simulink model "Grp43_Model"  (R2023a)
settings: Solver=FixedStepAuto  StartTime=0.0  StopTime=10.0  FixedStep=1e-5  RelTol=1e-3
values from neighbouring files (symbols this model uses):
  g = 9.8    [Grp43_Code.m]    (also in Grp43_part2_code.m = 9.81; e01 2.m; grp43_asgn2_2.m)
  l = 0.36    [Grp43_Code.m]    (also in Grp43_part2_code.m; e01 2.m; grp43_asgn2_2.m)
  m = 0.26    [Grp43_Code.m]    (also in Grp43_part2_code.m; e01 2.m; grp43_asgn2_2.m)
  M = 2.4    [Grp43_Code.m]    (also in Grp43_part2_code.m; e01 2.m; grp43_asgn2_2.m)
settings Model: Creator=jitbi  LastModifiedBy=Anirvan Krishna

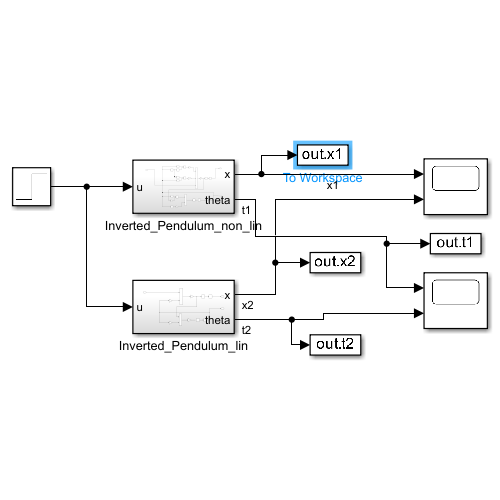
[thumbnail: Simulink's stored preview of the top-level diagram]
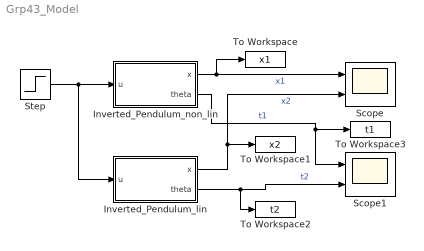
== system Grp43_Model ==
  Inverted_Pendulum_lin : Subsystem
  Inverted_Pendulum_non_lin : Subsystem
  Scope : Scope  NumInputPorts=2
  Scope1 : Scope  NumInputPorts=2
  Step : Step  Time=0
  To Workspace : ToWorkspace  VariableName=x1  SampleTime=-1
  To Workspace1 : ToWorkspace  VariableName=x2  SampleTime=-1
  To Workspace2 : ToWorkspace  VariableName=t2  SampleTime=-1
  To Workspace3 : ToWorkspace  VariableName=t1  SampleTime=-1
  wires:
  Step/1 -> Inverted_Pendulum_lin/1(u), Inverted_Pendulum_non_lin/1(u)
  Inverted_Pendulum_non_lin/1(x) -> Scope/1, To Workspace/1  "x1"
  Inverted_Pendulum_lin/1(x) -> To Workspace1/1, Scope/2  "x2"
  Inverted_Pendulum_non_lin/2(theta) -> To Workspace3/1, Scope1/1  "t1"
  Inverted_Pendulum_lin/2(theta) -> To Workspace2/1, Scope1/2  "t2"

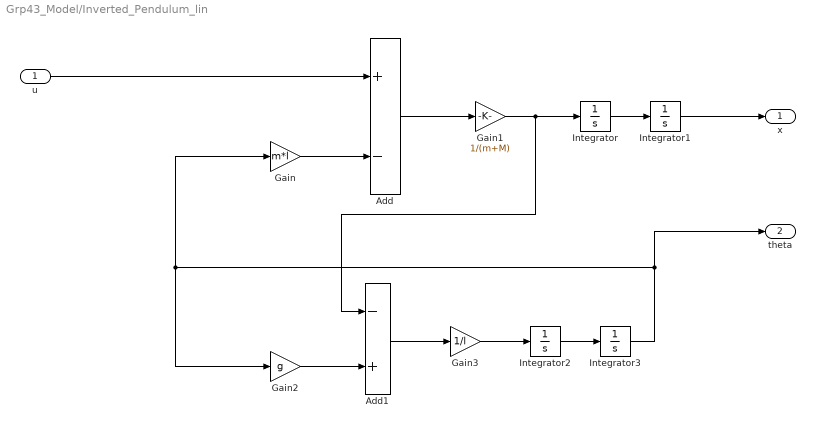
== system Grp43_Model/Inverted_Pendulum_lin ==
  u : Inport
  Add : Sum  Inputs=+-
  Add1 : Sum  Inputs=-+
  Gain : Gain  Gain=m*l
  Gain1 : Gain  Gain=1/(m+M)
  Gain2 : Gain  Gain=g
  Gain3 : Gain  Gain=1/l
  Integrator{,1..3} (4 alike) : Integrator
  x : Outport
  theta : Outport  Port=2
  wires:
  u/1 -> Add/1
  Gain/1 -> Add/2
  Integrator3/1 -> theta/1, Gain/1, Gain2/1
  Add/1 -> Gain1/1
  Integrator/1 -> Integrator1/1
  Gain1/1 -> Add1/1, Integrator/1
  Integrator1/1 -> x/1
  Gain2/1 -> Add1/2
  Add1/1 -> Gain3/1
  Integrator2/1 -> Integrator3/1
  Gain3/1 -> Integrator2/1

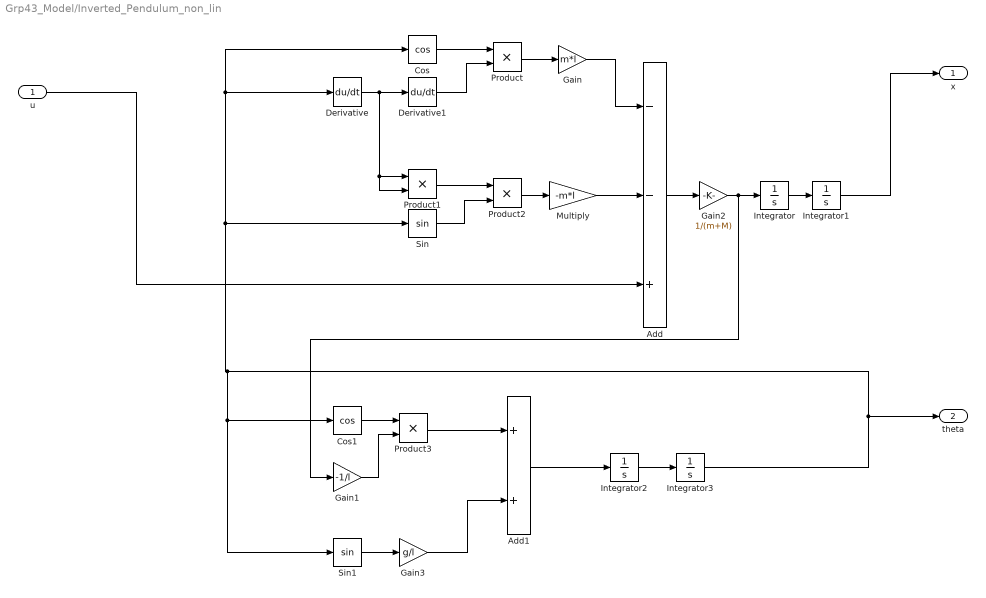
== system Grp43_Model/Inverted_Pendulum_non_lin ==
  u : Inport
  Add : Sum  Inputs=--+
  Add1 : Sum
  Cos : Trigonometry  Operator=cos
  Cos1 : Trigonometry  Operator=cos
  Derivative : Derivative
  Derivative1 : Derivative
  Gain : Gain  Gain=m*l
  Gain1 : Gain  Gain=-1/l
  Gain2 : Gain  Gain=1/(m+M)
  Gain3 : Gain  Gain=g/l
  Integrator{,1..3} (4 alike) : Integrator
  Multiply : Gain  Gain=-m*l
  Product{,1..3} (4 alike) : Product
  Sin : Trigonometry
  Sin1 : Trigonometry
  x : Outport
  theta : Outport  Port=2
  wires:
  Product2/1 -> Multiply/1
  Integrator3/1 -> Cos1/1, Sin1/1, Cos/1, Derivative/1, Sin/1, theta/1
  Add/1 -> Gain2/1
  Cos/1 -> Product/1
  Derivative/1 -> Product1/1, Product1/2, Derivative1/1
  u/1 -> Add/3
  Derivative1/1 -> Product/2
  Product/1 -> Gain/1
  Multiply/1 -> Add/2
  Integrator/1 -> Integrator1/1
  Gain2/1 -> Gain1/1, Integrator/1
  Product1/1 -> Product2/1
  Sin/1 -> Product2/2
  Gain/1 -> Add/1
  Integrator1/1 -> x/1
  Cos1/1 -> Product3/1
  Gain1/1 -> Product3/2
  Sin1/1 -> Gain3/1
  Product3/1 -> Add1/1
  Gain3/1 -> Add1/2
  Add1/1 -> Integrator2/1
  Integrator2/1 -> Integrator3/1
